simulink model "torqueBalancingTuning"  (Simulink 8.7)
settings: Solver=FixedStepDiscrete  StartTime=0.0  StopTime="CONFIG.SIMULATION_TIME "  FixedStep=CONFIG.Ts  RelTol=1e-3
InitFcn:
  | cd(fileparts(which(bdroot)));
  | initTorqueBalancing;
values from neighbouring files (symbols this model uses):
  baseToWorldRotationPort = ['/' WBT_modelName '/floatingBaseRotationMatrix:i']    [initTorqueBalancing.m]
  WBT_modelName = 'matlabTorqueBalancing'    [initTorqueBalancing.m]
undefined symbols (not defined in the file or in its folder): bVectorConstraints, CONFIG, ConstraintsMatrix, DiscIntNeverNeededParam, gain, references, reg, ROBOT_DOF, ROBOT_DOF_FOR_SIMULINK, sat, SM, sm, WBT_robotName
libraries: WBToolboxLibrary x171, simulink x11
(part 4 of 4)

== matlab function DesValues/LinearizationAndGainTuning/Subsystem/linearizationAndTuning ==
  data: qj input double; dqj input double; qjDes input double; ddqjLin output double; KSopt output double; KDopt output double; KSdes output double; KDdes output double; MomGain output double; intMomGain output double; xCoM input double; M input double; JG input double; JL input double; JR input double; w_H_l_sole input double; w_H_r_sole input double; LEFT_RIGHT_FOOT_IN_CONTACT input double; gain parameter double; reg parameter double; ROBOT_DOF_FOR_SIMULINK input double; KpNull output double; KdNull output double; ANull output double; BNull output double; Ax output double; Bx output double
function [ddqjLin,KSopt,KDopt,KSdes,KDdes,MomGain,intMomGain,KpNull,KdNull,ANull,BNull,Ax,Bx] = ...
          linearizeAndTuningFCN(qj,dqj,qjDes,xCoM,M,JG,JL,JR,w_H_l_sole,w_H_r_sole,LEFT_RIGHT_FOOT_IN_CONTACT,...
                                gain,reg,ROBOT_DOF_FOR_SIMULINK) 
%#codegen
Jc = [LEFT_RIGHT_FOOT_IN_CONTACT(1)*JL;
     LEFT_RIGHT_FOOT_IN_CONTACT(2)*JR];
  
  
[KpMom,KpNull,KdMom,KdNull,KS,KD,KSopt,KDopt,ANull,BNull,Ax,Bx,KSdes,KDdes]...
          = linearizeAndTuning(xCoM,M,JG,Jc,w_H_l_sole,w_H_r_sole,LEFT_RIGHT_FOOT_IN_CONTACT,gain,reg,ROBOT_DOF_FOR_SIMULINK);
                                                                               
% linearized joint accelerations     
ddqjLin    = -KS*(qj-qjDes)-KD*dqj; 

MomGain    = KdMom;
intMomGain = KpMom;
end
